simulink model "ensaio3"  (Simulink 6.0)
settings: Solver=ode45  StartTime=0.0  StopTime=10.0  RelTol=1e-3
values from neighbouring files (symbols this model uses):
  E = 9    [ensaio3.mat]
settings Model: Creator=ALUNO  LastModifiedBy=Andre
settings OptimizationCC: InlineInvariantSignals=off
settings DebuggingCC: SignalResolutionControl=UseLocalSettings
settings GRTTargetCC: TargetFcnLib=ansi_tfl_table_tmw.mat

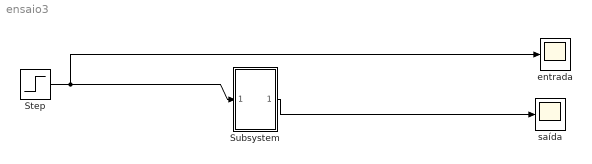
== system ensaio3 ==
  Step : Step  After=E  SampleTime=0
  Subsystem : Subsystem  mask{R=35.35, rg=1, b=0, fi=10, j=0.5, k=4}
  entrada : Scope
  saída : Scope
  wires:
  Step/1 -> entrada/1, Subsystem/1(In1)
  Subsystem/1(Out1) -> saída/1

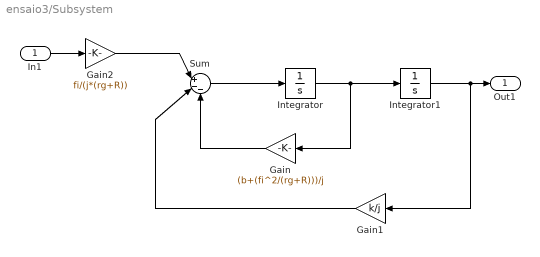
== system ensaio3/Subsystem ==
  In1 : Inport  Port=1  OutDataType=fixdt(1,16,0)  OutScaling=[]  LatchInput=off
  Gain : Gain  Orientation=left  Gain=(b+(fi^2/(rg+R)))/j
  Gain1 : Gain  Orientation=left  Gain=k/j
  Gain2 : Gain  Gain=fi/(j*(rg+R))
  Integrator : Integrator
  Integrator1 : Integrator
  Sum : Sum  Inputs=|+--
  Out1 : Outport  OutDataType=fixdt(1,16,0)  OutScaling=[]
  wires:
  Gain2/1 -> Sum/1
  Gain/1 -> Sum/3
  Gain1/1 -> Sum/2
  Sum/1 -> Integrator/1
  Integrator/1 -> Integrator1/1, Gain/1
  Integrator1/1 -> Gain1/1, Out1/1
  In1/1 -> Gain2/1
